simulink model "time"  (R2017b)
settings: Solver=FixedStepAuto  StartTime=0.0  StopTime=10.0  FixedStep=1  RelTol=1e-3
undefined symbols (not defined in the file): DiscIntNeverNeededParam
libraries: GPIO_Lib x6, TIMERS_Lib x3, USART_Lib x3, simulink x1
(part 2 of 2)

== system time/State Estimation and Complimentary Mixing/Subsystem1/Magnitude ==
  x_acc : Inport
  y_acc : Inport  Port=2
  z_acc : Inport  Port=3
  Demux1 : Demux  Outputs=3
  Math Function : Math  Operator=square  SaturateOnIntegerOverflow=on
  Mux : Mux  Inputs=3
  Sqrt : Sqrt  SaturateOnIntegerOverflow=on
  Sum : Sum  Inputs=+++
  |g| : Outport
  wires:
  Sqrt/1 -> |g|/1  "mag_acc"
  Sum/1 -> Sqrt/1
  Demux1/3 -> Sum/3
  Mux/1 -> Math Function/1
  Math Function/1 -> Demux1/1
  Demux1/1 -> Sum/1
  Demux1/2 -> Sum/2
  y_acc/1 -> Mux/2
  x_acc/1 -> Mux/1
  z_acc/1 -> Mux/3

== system time/Yaw/限幅到+-180/If Action Subsystem ==
  In1 : Inport
  Action Port : ActionPort
  Out1 : Outport
  wires:
  In1/1 -> Out1/1

== system time/Yaw/限幅到+-180/If Action Subsystem1 ==
  In1 : Inport
  Action Port : ActionPort
  Out1 : Outport
  wires:
  In1/1 -> Out1/1

== system time/Yaw/限幅到+-180/If Action Subsystem2 ==
  In1 : Inport
  Action Port : ActionPort
  Out1 : Outport
  wires:
  In1/1 -> Out1/1

== system time/Yaw/限幅到+-180，/If Action Subsystem ==
  In1 : Inport
  Action Port : ActionPort
  Out1 : Outport
  wires:
  In1/1 -> Out1/1

== system time/Yaw/限幅到+-180，/If Action Subsystem1 ==
  In1 : Inport
  Action Port : ActionPort
  Out1 : Outport
  wires:
  In1/1 -> Out1/1

== system time/Yaw/限幅到+-180，/If Action Subsystem2 ==
  In1 : Inport
  Action Port : ActionPort
  Out1 : Outport
  wires:
  In1/1 -> Out1/1

== system time/Yaw/限幅到+-180，，/If Action Subsystem ==
  In1 : Inport
  Action Port : ActionPort
  Out1 : Outport
  wires:
  In1/1 -> Out1/1

== system time/Yaw/限幅到+-180，，/If Action Subsystem1 ==
  In1 : Inport
  Action Port : ActionPort
  Out1 : Outport
  wires:
  In1/1 -> Out1/1

== system time/Yaw/限幅到+-180，，/If Action Subsystem2 ==
  In1 : Inport
  Action Port : ActionPort
  Out1 : Outport
  wires:
  In1/1 -> Out1/1

== stateflow chart time/PWM/Subsystem1/Chart1 ==
  (default) -> (junction 4)
  (junction 4) -> (junction 6) : {ANO_DT_Send_MotoPWM(m_1,m_2,m_3,m_4,0,0,0,0);}
  data: m_1 input; m_2 input; m_3 input; m_4 input

== stateflow chart time/Subsystem/Chart1 ==
  (default) -> (junction 4)
  (junction 4) -> (junction 6) : {ANO_DT_Send_Status(roll, pitch, yaw,0,0,0);}
  data: roll input single size=1; pitch input single size=1; yaw input single size=1

== stateflow chart time/Chart ==
  note: 
  note: 第一步设置动作语言为C语言
  note: 如果做上电进行陀螺仪和加速度校准的话，可以在循环执行上面做个校准的simulink函数，然后辅助可以做下按键执行传感器校准,并进行上电校准判断是否处于运动的过程中
  state start
    entry:y=1;
    du:i=i+1
  (default) -> start
  start -> start : {y=0;}
  data: i local int8 size=1 =0; y output double

== matlab function time/pwm_out1 ==
  data: Roll input; M1 output; Pitch input; Yaw input; Thrust input; M2 output; M3 output; M4 output
function [M1, M2, M3, M4] = motor_mixer(Roll, Pitch, Yaw, Thrust)

% idle_PWM = uint16(1000);

% Quad X
M1 = ((Roll - Pitch - Yaw) / 2 * Thrust + Thrust) ;
M2 = ((-Roll - Pitch + Yaw) / 2 * Thrust + Thrust) ;
M3 = ((-Roll + Pitch - Yaw) / 2 * Thrust + Thrust) ;
M4 = ((Roll + Pitch + Yaw) / 2 * Thrust + Thrust);
% M5 = 1000;
% M6 = 1000;
% M7 = 1000;
% M8 = 1000;

% Quad +
% M1 = ((Pitch - Yaw) * Thrust / 2 + Thrust) * 1000 + idle_PWM;
% M2 = ((-Roll + Yaw) * Thrust / 2 + Thrust) * 1000 + idle_PWM;
% M3 = ((-Pitch - Yaw) * Thrust / 2 + Thrust) * 1000 + idle_PWM;
% M4 = ((Roll + Yaw) * Thrust / 2 + Thrust) * 1000 + idle_PWM;
% M5 = 1000;
% M6 = 1000;
% M7 = 1000;
% M8 = 1000;

% Hex X
% M1 = ((Pitch + Roll / 2 - Yaw) * Thrust / 2 + Thrust) * 1000 + idle_PWM;
% M2 = ((Pitch - Roll / 2 + Yaw) * Thrust / 2 + Thrust) * 1000 + idle_PWM;
% M3 = ((-Roll - Yaw) * Thrust / 2 + Thrust) * 1000 + idle_PWM;
% M4 = ((-Pitch - Roll / 2 + Yaw) * Thrust / 2 + Thrust) * 1000 + idle_PWM;
% M5 = ((-Pitch + Roll / 2 - Yaw) * Thrust / 2 + Thrust) * 1000 + idle_PWM;
% M6 = ((Roll + Yaw) * Thrust / 2 + Thrust) * 1000 + idle_PWM;
% M7 = 1000;
% M8 = 1000;

% Hex X (From Adam)
% M1 = uint16(single(((-Roll - Yaw) * Thrust / 3 + Thrust) * single(1000))) + idle_PWM;
% M2 = uint16(single(((Roll + Yaw) * Thrust / 3 + Thrust) * single(1000))) + idle_PWM;
% M3 = uint16(single(((Pitch + (Roll / 2) - Yaw) * Thrust / 3 + Thrust) * single(1000))) + idle_PWM;
% M4 = uint16(single(((-Pitch - (Roll / 2) + Yaw) * Thrust / 3 + Thrust) * single(1000))) + idle_PWM;
% M5 = uint16(single(((Pitch - (Roll / 2) + Yaw) * Thrust / 3 + Thrust) * single(1000))) + idle_PWM;
% M6 = uint16(single(((-Pitch + (Roll / 2) - Yaw) * Thrust / 3 + Thrust) * single(1000))) + idle_PWM;

% Hex X (Version 2)
% Roll/Yaw
% M1 = ((-Roll - Yaw) * Thrust / 2 + Thrust) * 1000 + idle_PWM;
% M2 = ((Roll + Yaw) * Thrust / 2 + Thrust) * 1000 + idle_PWM;
% % + Pitch/Roll
% M6 = ((Pitch + Roll / 2 - Yaw) * Thrust / 2 + Thrust) * 1000 + idle_PWM;
% M4 = ((Pitch - Roll / 2 + Yaw) * Thrust / 2 + Thrust) * 1000 + idle_PWM;
% % - Pitch/Roll
% M5 = ((-Pitch - Roll / 2 + Yaw) * Thrust / 2 + Thrust) * 1000 + idle_PWM;
% M3 = ((-Pitch + Roll / 2 - Yaw) * Thrust / 2 + Thrust) * 1000 + idle_PWM;

== stateflow chart time/Chart1 ==
  state offset=calOffset(gyro_x,gyro_y,gyro_z,acc_x,acc_y,acc_z) [function]
  (default) -> (junction 16) : /* calOffset */
  (junction 16) -> (junction 17) [order 1] : [i<200]
  (junction 16) -> (junction 18) [order 2] : [i>=200]
  (junction 17) -> (junction 19) : {i++;offset=calOffset(gx,gy,gz,ax,ay,az);}
  (junction 19) -> (junction 18)
  (junction 18) -> (junction 20)
  data: gyro_x function_input int32; gyro_y function_input int32; gyro_z function_input int32; acc_x function_input int32; acc_y function_input int32; acc_z function_input int32; offset function_output single; ax input int32; ay input int32; az input int32; gx input int32; gy input int32; gz input int32; i local int16 size=1 =0; offset output int32 size=6*1

== matlab function time/Subsystem5/CHAR convertion1 ==
  data: u1 input; NbChar output uint16 size=1; Buff output uint32 size=1; u2 input; u3 input; u4 input
function [NbChar, Buff] = convert(u1,u2,u3,u4)
if coder.target('Sfun')
% Executing in MATLAB, Buff is null
Buff = uint32(0);
NbChar = uint16(0);
else
buffer = zeros(1,51,'uint8');
% tmp1=u1*57.3;
% tmp2=u2*57.3;
% tmp3=u3*57.3;
coder.ceval('sprintf',coder.wref(buffer),['%f %f %f %f', 13, 10, 0],u1,u2,u3,u4);
Buff = coder.ceval('getBuffPtr',coder.wref(buffer));
NbChar =coder.ceval('strlen',coder.ref(buffer));
end
end

== matlab function time/Subsystem1/CHAR convertion1 ==
  data: u1 input; NbChar output uint16 size=1; Buff output uint32 size=1; u2 input; u3 input; u4 input
function [NbChar, Buff] = convert(u1,u2,u3,u4)
if coder.target('Sfun')
% Executing in MATLAB, Buff is null
Buff = uint32(0);
NbChar = uint16(0);
else
buffer = zeros(1,51,'uint8');
% tmp1=u1*57.3;
% tmp2=u2*57.3;
% tmp3=u3*57.3;
coder.ceval('sprintf',coder.wref(buffer),['%f %f %f %f', 13, 10, 0],u1,u2,u3,u4);
Buff = coder.ceval('getBuffPtr',coder.wref(buffer));
NbChar =coder.ceval('strlen',coder.ref(buffer));
end
end

== matlab function time/Yaw/CHAR convertion ==
  data: u1 input; NbChar output uint16 size=1; Buff output uint32 size=1; u2 input
function [NbChar, Buff] = convert(u1,u2)
if coder.target('Sfun')
% Executing in MATLAB, Buff is null
Buff = uint32(0);
NbChar = uint16(0);
else
buffer = zeros(1,51,'uint8');
% tmp1=u1*57.3;
% tmp2=u2*57.3;
% tmp3=u3*57.3;
coder.ceval('sprintf',coder.wref(buffer),['%f %f', 13, 10, 0],u1,u2);
Buff = coder.ceval('getBuffPtr',coder.wref(buffer));
NbChar =coder.ceval('strlen',coder.ref(buffer));
end
end

== stateflow chart time/Chart2 ==
  note: 
  note: 第一步设置动作语言为C语言
  state start
    entry:
    receiveData(rcDataTmp);
    checkLock();
    du:i=i+1
  state middle
    du:i=i+1
  state checkLock [function]
    (default) -> (junction 62)
    (junction 62) -> (junction 63) [order 1] : [FlyOk==0&&(rcDataTmp[2]<1100)&&(rcDataTmp[3]>1900)]{OpenLock=OpenLock+1}
    (junction 63) -> (junction 65) : [OpenLock>100]{FlyOk=1;OpenLock=100;}
    (junction 62) -> (junction 64) [order 2] : [FlyOk==1&&(rcDataTmp[2]<1100)&&(rcDataTmp[3]<1100)]{OpenLock=OpenLock-1}
    (junction 64) -> (junction 66) : [OpenLock<0]{OpenLock=0;FlyOk=0;}
  (default) -> start : {NRF24L01_SPI_Init();}
  start -> middle : [i>5]{i=0;}
  middle -> start : [i>5]{i=0;}
  data: rcDataTmp output uint16 size=4*1 =0; OpenLock local int16 size=1 =0; FlyOk output int8 size=1 =0; i local int8

== stateflow chart time/Chart3 ==
  note: 
  note: 第一步设置动作语言为C语言
  note: 如果做上电进行陀螺仪和加速度校准的话，可以在循环执行上面做个校准的simulink函数，然后辅助可以做下按键执行传感器校准,并进行上电校准判断是否处于运动的过程中
  state start
    entry:i=i+1;MPU6050ReadGyro(gyroData);
    MPU6050ReadAcc(accData);
    ANO_DT_Send_Senser(accData[0],accData[1],accData[2],gyroData[0],gyroData[1],gyroData[2],0,0,0,0);
  state middle
    du:i=i+1;
  (default) -> start
  start -> middle : after(2,tick)
  middle -> start : after(2,tick)
  data: gyroData output int16 size=3*1 =0; accData output int16 size=3*1 =0; i local int8 size=1 =0

== stateflow chart time/Chart4 ==
  state pwmInit [function]
  (default) -> (junction 16) : /* init */
  (junction 16) -> (junction 17) [order 1] : [i<1]
  (junction 16) -> (junction 18) [order 2] : [i>=1]
  (junction 17) -> (junction 19) : {i++;pwmInit();I2C_InitGPIO();MPU6050_Init();}
  (junction 19) -> (junction 18)
  (junction 18) -> (junction 20)
  data: i local int8 size=1 =0

== stateflow chart time/Chart9 ==
  note: 
  state pwmInit [function]
  note: 第一步设置动作语言为C语言
  note: 如果做上电进行陀螺仪和加速度校准的话，可以在循环执行上面做个校准的simulink函数，然后辅助可以做下按键执行传感器校准,并进行上电校准判断是否处于运动的过程中
  state start
    entry:MPU6050ReadGyro(gyroData);
    MPU6050ReadAcc(accData);
    ANO_DT_Send_Senser(accData[0],accData[1],accData[2],gyroData[0],gyroData[1],gyroData[2],0,0,0,0);
    du:i=i+1
  state middle
    du:i=i+1;
  (default) -> start : {pwmInit();I2C_InitGPIO();MPU6050_Init();}
  start -> middle : [i>4]{i=0;}
  middle -> start : [i>4]{i=0;}
  data: gyroData output int16 size=3*1 =0; accData output int16 size=3*1 =0; i local int8 size=1 =0
